simulink model "sampleModel1916"  (R2023a)
settings: Solver=VariableStepAuto  StartTime=0.0  StopTime=10.0  RelTol=1e-3
libraries: hdlsllib x5, simulink x1
settings Model: Creator=user1  LastModifiedBy=user1

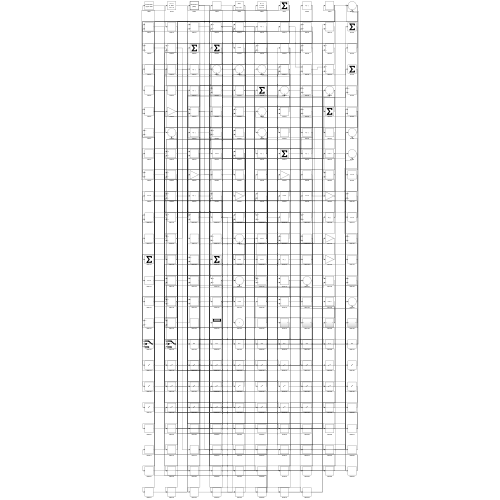
[thumbnail: Simulink's stored preview of the top-level diagram]
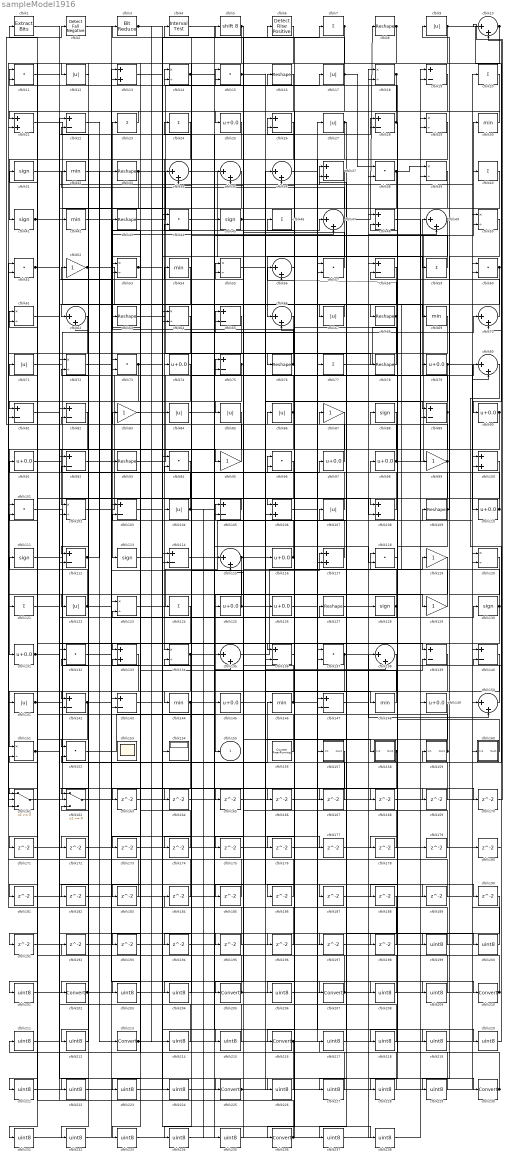
== system sampleModel1916 ==
  cfblk1 : simulink/Logic and Bit Operations/Extract Bits  bitsToExtract=Upper half  numBits=8  bitIdxRange=[0 7]  outScalingMode=Preserve fixed-point scaling
      settings: LibrarySourceBlock=|
      | hdlsllib/Logic and Bit
      | Operations/Extract Bits
  cfblk{10,34..36,47,49,56,62,66,70,80,115,135,138,150} (15 alike) : Sum  Inputs=|++
  cfblk{13,21,37,48,100,106,108,117,133} (9 alike) : Sum
  cfblk{11,15,38,44,51,57,60,73,94,96,101,118,132,137,152} (15 alike) : DotProduct  OutDataTypeStr=Inherit: Inherit via internal rule
  cfblk{14,18,29,39,50,53,55,61,64,72,102,120,123,134,151} (15 alike) : Product  Inputs=*/  RndMeth=Zero  SaturateOnIntegerOverflow=on
  cfblk{19,22,26,28,58,65,75,81..82,89,92,103,105,112,114,136,139..140,142..143,147} (21 alike) : Sum  Inputs=+-
  cfblk{9,12,17,27,67,71,84..86,104,107,122,141} (13 alike) : Abs  SaturateOnIntegerOverflow=off
  cfblk{8,16,33,43,63,68,76,78,93,109,127} (11 alike) : Reshape
  cfblk{25,74,79,90..91,97..98,110,116,125..126,131,145,149} (14 alike) : Bias  Bias=0.0  SaturateOnIntegerOverflow=off
  cfblk{31,41,45,88,111,113,128,130} (8 alike) : Signum
  cfblk{52,83,87,95,99,119,129} (7 alike) : Gain
  cfblk{7,20,23..24,40,46,59,77,121,124} (10 alike) : Sum  Inputs=+
  cfblk{30,32,42,54,69,144,146,148} (8 alike) : MinMax
  cfblk153 : Scope
      settings: Floating=on
  cfblk154 : Display
  cfblk156 : hdlsllib/Sources/Counter Free-Running  NumBits=16  tsamp=-1
  cfblk157 : Subsystem
      settings: LibrarySourceBlock=|
      | hdlsllib/Ports &
      | Subsystems/Subsystem
  cfblk158 : Subsystem
      settings: LibrarySourceBlock=|
      | hdlsllib/Ports &
      | Subsystems/Subsystem
  cfblk159 : Subsystem
      settings: LibrarySourceBlock=|
      | hdlsllib/Ports &
      | Subsystems/Subsystem
  cfblk160 : Subsystem
      settings: LibrarySourceBlock=|
      | hdlsllib/Ports &
      | Subsystems/Subsystem
  cfblk161 : Switch  SaturateOnIntegerOverflow=off  InputSameDT=off
  cfblk162 : Switch  SaturateOnIntegerOverflow=off  InputSameDT=off
  cfblk{163..198} (36 alike) : Delay  SampleTime=1
  cfblk{199..201,203..204,206,208..209,211..212,214..215,217..224,226..229,231..235,237..238} (31 alike) : DataTypeConversion  OutDataTypeStr=uint8  SaturateOnIntegerOverflow=off  RndMeth=Floor
  cfblk2 : hdlsllib/Logic and Bit Operations/Detect Fall Negative  vinit=0  OutDataTypeStr=boolean
  cfblk{202,205,207,210,213,216,225,230,236} (9 alike) : DataTypeConversion  SaturateOnIntegerOverflow=off  RndMeth=Floor
  cfblk3 : hdlsllib/Logic and Bit Operations/Bit Reduce  mode=AND
  cfblk4 : hdlsllib/Logic and Bit Operations/Interval Test  IntervalClosedRight=on  uplimit=0.5  IntervalClosedLeft=on  lowlimit=-0.5  OutDataTypeStr=boolean
  cfblk5 : ArithShift  BitShiftNumber=8
  cfblk6 : hdlsllib/Logic and Bit Operations/Detect Rise Positive  vinit=0  OutDataTypeStr=boolean
  cfblk155 : Outport  VectorParamsAs1DForOutWhenUnconnected=off
  wires:
  cfblk68/1 -> cfblk56/2, cfblk185/1, cfblk186/1
  cfblk77/1 -> cfblk16/1
  cfblk95/1 -> cfblk2/1
  cfblk139/1 -> cfblk155/1
  cfblk6/1 -> cfblk81/1
  cfblk63/1 -> cfblk134/1
  cfblk101/1 -> cfblk146/1
  cfblk60/1 -> cfblk105/1, cfblk76/1
  cfblk22/1 -> cfblk213/1
  cfblk24/1 -> cfblk74/1
  cfblk42/1 -> cfblk113/1
  cfblk133/1 -> cfblk151/1
  cfblk119/1 -> cfblk145/1
  cfblk151/1 -> cfblk195/1, cfblk196/1
  cfblk93/1 -> cfblk49/1
  cfblk49/1 -> cfblk66/1, cfblk176/1
  cfblk97/1 -> cfblk71/1
  cfblk23/1 -> cfblk21/1
  cfblk141/1 -> cfblk96/1, cfblk101/2, cfblk127/1
  cfblk135/1 -> cfblk119/1
  cfblk149/1 -> cfblk205/1
  cfblk102/1 -> cfblk80/1
  cfblk113/1 -> cfblk7/1
  cfblk8/1 -> cfblk12/1, cfblk173/1
  cfblk134/1 -> cfblk144/1, cfblk26/1
  cfblk13/1 -> cfblk230/1
  cfblk76/1 -> cfblk23/1, cfblk34/2
  cfblk127/1 -> cfblk49/2
  cfblk3/1 -> cfblk154/1, cfblk84/1, cfblk59/1
  cfblk25/1 -> cfblk104/1
  cfblk98/1 -> cfblk30/1, cfblk37/2
  cfblk9/1 -> cfblk90/1, cfblk21/2, cfblk162/1, cfblk161/2
  cfblk111/1 -> cfblk79/1
  cfblk130/1 -> cfblk46/1, cfblk142/2
  cfblk159/1(Out1) -> cfblk107/1, cfblk26/2
  cfblk82/1 -> cfblk131/1
  cfblk136/1 -> cfblk6/1
  cfblk67/1 -> cfblk62/1
  cfblk80/1 -> cfblk159/1(In1)
  cfblk104/1 -> cfblk91/1, cfblk118/2, cfblk235/1
  cfblk56/1 -> cfblk66/2
  cfblk123/1 -> cfblk77/1
  cfblk45/1 -> cfblk138/2, cfblk148/1
  cfblk48/1 -> cfblk99/1
  cfblk75/1 -> cfblk85/1, cfblk93/1
  cfblk19/1 -> cfblk236/1
  cfblk142/1 -> cfblk117/1, cfblk190/1, cfblk191/1
  cfblk146/1 -> cfblk15/1, cfblk220/1
  cfblk122/1 -> cfblk111/1, cfblk47/2
  cfblk112/1 -> cfblk62/2, cfblk33/1
  cfblk30/1 -> cfblk25/1
  cfblk108/1 -> cfblk55/1
  cfblk162/1 -> cfblk10/1
  cfblk47/1 -> cfblk8/1, cfblk117/2, cfblk32/1
  cfblk158/1(Out1) -> cfblk193/1, cfblk194/1
  cfblk16/1 -> cfblk135/1
  cfblk61/1 -> cfblk40/1
  cfblk137/1 -> cfblk150/2, cfblk162/2
  cfblk145/1 -> cfblk97/1
  cfblk43/1 -> cfblk17/1
  cfblk109/1 -> cfblk9/1, cfblk61/1, cfblk198/1
  cfblk64/1 -> cfblk81/2
  cfblk105/1 -> cfblk103/1
  cfblk34/1 -> cfblk137/2
  cfblk71/1 -> cfblk65/1
  cfblk57/1 -> cfblk15/2
  cfblk79/1 -> cfblk110/1, cfblk106/2
  cfblk106/1 -> cfblk157/1(In1)
  cfblk161/1 -> cfblk37/1
  cfblk38/1 -> cfblk39/1, cfblk206/1
  cfblk90/1 -> cfblk102/1, cfblk106/1
  cfblk99/1 -> cfblk36/2, cfblk161/1
  cfblk29/1 -> cfblk114/2
  cfblk5/1 -> cfblk164/1, cfblk165/1
  cfblk160/1(Out1) -> cfblk118/1
  cfblk115/1 -> cfblk158/1(In1), cfblk161/3
  cfblk110/1 -> cfblk98/1, cfblk56/1
  cfblk91/1 -> cfblk55/2
  cfblk39/1 -> cfblk68/1
  cfblk116/1 -> cfblk63/1, cfblk44/2
  cfblk131/1 -> cfblk130/1, cfblk189/1
  cfblk65/1 -> cfblk143/2
  cfblk46/1 -> cfblk136/1
  cfblk18/1 -> cfblk152/1, cfblk141/1
  cfblk31/1 -> cfblk69/1
  cfblk117/1 -> cfblk75/1
  cfblk92/1 -> cfblk210/1
  cfblk26/1 -> cfblk41/1
  cfblk121/1 -> cfblk42/1
  cfblk33/1 -> cfblk78/1, cfblk232/1
  cfblk94/1 -> cfblk202/1
  cfblk27/1 -> cfblk57/2, cfblk167/1, cfblk201/1
  cfblk21/1 -> cfblk64/2
  cfblk148/1 -> cfblk83/1
  cfblk36/1 -> cfblk147/2
  cfblk52/1 -> cfblk67/1, cfblk47/1
  cfblk129/1 -> cfblk52/1
  cfblk15/1 -> cfblk126/1, cfblk89/1
  cfblk10/1 -> cfblk121/1, cfblk212/1
  cfblk37/1 -> cfblk133/1, cfblk112/2
  cfblk14/1 -> cfblk129/1, cfblk139/1
  cfblk53/1 -> cfblk209/1, cfblk214/1
  cfblk107/1 -> cfblk11/1
  cfblk114/1 -> cfblk60/2
  cfblk144/1 -> cfblk50/2, cfblk139/2, cfblk163/1
  cfblk41/1 -> cfblk136/2, cfblk28/1
  cfblk152/1 -> cfblk45/1
  cfblk54/1 -> cfblk102/2
  cfblk147/1 -> cfblk18/1
  cfblk7/1 -> cfblk51/2, cfblk112/1, cfblk142/1
  cfblk69/1 -> cfblk122/1
  cfblk89/1 -> cfblk54/1, cfblk204/1
  cfblk150/1 -> cfblk88/1
  cfblk84/1 -> cfblk75/2
  cfblk17/1 -> cfblk5/1, cfblk38/1, cfblk34/1, cfblk115/2
  cfblk28/1 -> cfblk14/1, cfblk178/1
  cfblk156/1 -> cfblk31/1
  cfblk73/1 -> cfblk28/2, cfblk181/1, cfblk182/1
  cfblk125/1 -> cfblk109/1, cfblk14/2
  cfblk72/1 -> cfblk207/1
  cfblk70/1 -> cfblk48/2
  cfblk128/1 -> cfblk123/2, cfblk3/1
  cfblk59/1 -> cfblk4/1
  cfblk40/1 -> cfblk53/1
  cfblk78/1 -> cfblk11/2
  cfblk87/1 -> cfblk216/1
  cfblk132/1 -> cfblk70/1
  cfblk51/1 -> cfblk53/2, cfblk108/1, cfblk108/2
  cfblk81/1 -> cfblk95/1
  cfblk1/1 -> cfblk225/1
  cfblk86/1 -> cfblk24/1, cfblk125/1
  cfblk164/1 -> cfblk134/2
  cfblk165/1 -> cfblk18/2
  cfblk88/1 -> cfblk166/1
  cfblk166/1 -> cfblk150/1
  cfblk167/1 -> cfblk152/2
  cfblk126/1 -> cfblk168/1
  cfblk168/1 -> cfblk29/1
  cfblk11/1 -> cfblk169/1
  cfblk169/1 -> cfblk143/1
  cfblk2/1 -> cfblk170/1
  cfblk170/1 -> cfblk10/2
  cfblk62/1 -> cfblk171/1
  cfblk171/1 -> cfblk36/1
  cfblk12/1 -> cfblk172/1
  cfblk172/1 -> cfblk80/2
  cfblk85/1 -> cfblk174/1
  cfblk174/1 -> cfblk103/2
  cfblk66/1 -> cfblk175/1
  cfblk175/1 -> cfblk48/1
  cfblk176/1 -> cfblk89/2
  cfblk32/1 -> cfblk177/1
  cfblk177/1 -> cfblk138/1
  cfblk178/1 -> cfblk105/2
  cfblk179/1 -> cfblk57/1
  cfblk180/1 -> cfblk70/2
  cfblk181/1 -> cfblk65/2
  cfblk100/1 -> cfblk183/1
  cfblk183/1 -> cfblk123/1
  cfblk184/1 -> cfblk132/2
  cfblk185/1 -> cfblk51/1
  cfblk186/1 -> cfblk162/3
  cfblk55/1 -> cfblk187/1
  cfblk187/1 -> cfblk50/1
  cfblk118/1 -> cfblk188/1
  cfblk189/1 -> cfblk82/1
  cfblk191/1 -> cfblk135/2
  cfblk192/1 -> cfblk38/2
  cfblk193/1 -> cfblk147/1
  cfblk194/1 -> cfblk115/1
  cfblk195/1 -> cfblk114/1
  cfblk196/1 -> cfblk133/2
  cfblk4/1 -> cfblk197/1
  cfblk197/1 -> cfblk60/1
  cfblk198/1 -> cfblk86/1
  cfblk120/1 -> cfblk199/1
  cfblk199/1 -> cfblk101/1
  cfblk182/1 -> cfblk200/1
  cfblk200/1 -> cfblk120/1
  cfblk201/1 -> cfblk120/2
  cfblk202/1 -> cfblk180/1, cfblk179/1, cfblk64/1
  cfblk157/1(Out1) -> cfblk203/1
  cfblk203/1 -> cfblk94/1
  cfblk204/1 -> cfblk94/2
  cfblk205/1 -> cfblk61/2, cfblk137/1
  cfblk206/1 -> cfblk149/1
  cfblk207/1 -> cfblk184/1, cfblk39/2
  cfblk83/1 -> cfblk208/1
  cfblk208/1 -> cfblk72/1
  cfblk209/1 -> cfblk72/2
  cfblk210/1 -> cfblk192/1, cfblk82/2
  cfblk211/1 -> cfblk92/1
  cfblk212/1 -> cfblk92/2
  cfblk213/1 -> cfblk100/1, cfblk27/1
  cfblk214/1 -> cfblk22/1
  cfblk173/1 -> cfblk215/1
  cfblk215/1 -> cfblk22/2
  cfblk216/1 -> cfblk211/1, cfblk160/1(In1)
  cfblk217/1 -> cfblk87/1
  cfblk140/1 -> cfblk218/1
  cfblk218/1 -> cfblk73/1
  cfblk44/1 -> cfblk219/1
  cfblk219/1 -> cfblk140/1
  cfblk220/1 -> cfblk140/2
  cfblk124/1 -> cfblk221/1
  cfblk221/1 -> cfblk73/2
  cfblk96/1 -> cfblk222/1
  cfblk222/1 -> cfblk124/1
  cfblk20/1 -> cfblk223/1
  cfblk223/1 -> cfblk116/1
  cfblk143/1 -> cfblk224/1
  cfblk224/1 -> cfblk20/1
  cfblk225/1 -> cfblk100/2, cfblk29/2
  cfblk163/1 -> cfblk226/1
  cfblk226/1 -> cfblk1/1
  cfblk58/1 -> cfblk227/1
  cfblk227/1 -> cfblk43/1
  cfblk190/1 -> cfblk228/1
  cfblk228/1 -> cfblk58/1
  cfblk50/1 -> cfblk229/1
  cfblk229/1 -> cfblk58/2
  cfblk230/1 -> cfblk217/1, cfblk44/1
  cfblk74/1 -> cfblk231/1
  cfblk231/1 -> cfblk13/1
  cfblk232/1 -> cfblk13/2
  cfblk35/1 -> cfblk233/1
  cfblk233/1 -> cfblk128/1
  cfblk138/1 -> cfblk234/1
  cfblk234/1 -> cfblk35/1
  cfblk235/1 -> cfblk35/2
  cfblk236/1 -> cfblk96/2, cfblk151/2, cfblk132/1
  cfblk188/1 -> cfblk237/1
  cfblk237/1 -> cfblk19/1
  cfblk103/1 -> cfblk238/1
  cfblk238/1 -> cfblk19/2

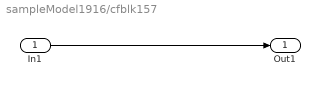
== system sampleModel1916/cfblk157 ==
  In1 : Inport
  Out1 : Outport
  wires:
  In1/1 -> Out1/1

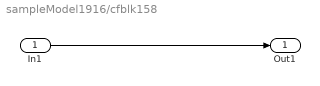
== system sampleModel1916/cfblk158 ==
  In1 : Inport
  Out1 : Outport
  wires:
  In1/1 -> Out1/1

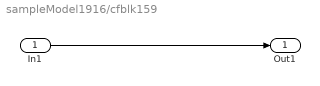
== system sampleModel1916/cfblk159 ==
  In1 : Inport
  Out1 : Outport
  wires:
  In1/1 -> Out1/1

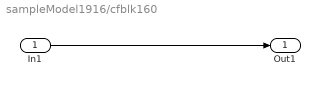
== system sampleModel1916/cfblk160 ==
  In1 : Inport
  Out1 : Outport
  wires:
  In1/1 -> Out1/1
